simulink model "Final_Reciprocating_Simscape_Impedance_Hybrid_01_09_24_1_Pos"  (R2023b)
settings: Solver=VariableStepAuto  StartTime=0.0  StopTime=0.5  RelTol=1e-3
values from neighbouring files (symbols this model uses):
  d1 = 0    [FFFB_PosForce_ME1.m]    (also in FFFB_PosForce_ME2.m; FFFB_Posarbitary_actual_Mass.m; FFFB_arbitary_actual_Mass.m; Kin_sol_Pos2.m)
  d2 = 0    [FFFB_PosForce_ME1.m]    (also in FFFB_PosForce_ME2.m; FFFB_Posarbitary_actual_Mass.m; FFFB_arbitary_actual_Mass.m; Kin_sol_Pos2.m)
  k1 = 20    [FFFB_PosForce_ME1.m]    (also in FFFB_PosForce_ME2.m; FFFB_Posarbitary_actual_Mass.m; FFFB_arbitary_actual_Mass.m; KinAnimation_plot.m = double(a11*cos(f)*cos(t1+t2)-b11*sin(f)*sin(t1+t2)+P31(1)))
  k2 = 4    [FFFB_PosForce_ME1.m]    (also in FFFB_PosForce_ME2.m; FFFB_Posarbitary_actual_Mass.m; FFFB_arbitary_actual_Mass.m; KinAnimation_plot.m = double(a11*cos(f)*sin(t1+t2)+b11*sin(f)*cos(t1+t2)+P31(2)))
  Kd = 0.5    [FFFB_PosForce_ME.m]    (also in FFFB_PosForce_ME1.m = 2.8284; FFFB_PosForce_ME2.m = 2.8284; FFFB_Posarbitary_actual_Mass.m = 2.8284; FFFB_arbitary_actual_Mass.m = 2.8284)
  Kd1 = 1    [FFFB_PosForce_ME.m]    (also in FFFB_PosForce_ME1.m = 141.42; FFFB_PosForce_ME2.m = 141.42; FFFB_Posarbitary_actual_Mass.m = 141.42; FFFB_arbitary_actual_Mass.m = 141.42)
  Kd2 = 110    [FFFB_PosForce_ME1.m]    (also in FFFB_PosForce_ME2.m; FFFB_Posarbitary_actual_Mass.m; FFFB_arbitary_actual_Mass.m; Kin_sol_Pos2.m)
  Kp = 16    [FFFB_PosForce_ME.m]    (also in FFFB_PosForce_ME1.m = 2; FFFB_PosForce_ME2.m = 2; FFFB_Posarbitary_actual_Mass.m = 2; FFFB_arbitary_actual_Mass.m = 2)
  Kp1 = 10    [FFFB_PosForce_ME.m]    (also in FFFB_PosForce_ME1.m = 5000; FFFB_PosForce_ME2.m = 5000; FFFB_Posarbitary_actual_Mass.m = 5000; FFFB_arbitary_actual_Mass.m = 5000)
  Kp2 = 10000    [FFFB_PosForce_ME1.m]    (also in FFFB_PosForce_ME2.m; FFFB_Posarbitary_actual_Mass.m; FFFB_arbitary_actual_Mass.m; Kin_Trajectory_23_09_24.m)
  m1 = 0.6562    [FFFB_PosForce_ME1.m]    (also in FFFB_PosForce_ME2.m; FFFB_Posarbitary_actual_Mass.m; FFFB_arbitary_actual_Mass.m; Kin_sol_Pos2.m)
  m2 = 0.1355    [FFFB_PosForce_ME1.m]    (also in FFFB_PosForce_ME2.m; FFFB_Posarbitary_actual_Mass.m; FFFB_arbitary_actual_Mass.m; Kin_sol_Pos2.m)
  m3 = 0.1336    [FFFB_PosForce_ME1.m]    (also in FFFB_PosForce_ME2.m; FFFB_Posarbitary_actual_Mass.m; FFFB_arbitary_actual_Mass.m; Kin_sol_Pos2.m)
  N = [-y1+y3;-x3+x1]    [Contact.m]
  P = [X2';Y2';F2']    [FFFB_PosForce_ME.m]    (also in FFFB_PosForce_ME1.m = [X;Y;F_]; FFFB_PosForce_ME2.m = [X;Y;F_]; FFFB_Posarbitary_actual_Mass.m = [X;Y;F_]; FFFB_arbitary_actual_Mass.m = [X;Y;F_])
  Pd = [Xd2';Yd2';Fd2']    [FFFB_PosForce_ME.m]    (also in FFFB_PosForce_ME1.m = [Xd;Yd;Fd_]; FFFB_PosForce_ME2.m = [Xd;Yd;Fd_]; FFFB_Posarbitary_actual_Mass.m = [Xd;Yd;Fd_]; FFFB_arbitary_actual_Mass.m = [Xd;Yd;Fd_])
  Pdd = [Xdd2';Ydd2';Fdd2']    [FFFB_PosForce_ME.m]    (also in FFFB_PosForce_ME1.m = [Xdd;Ydd;Fdd_]; FFFB_PosForce_ME2.m = [Xdd;Ydd;Fdd_]; FFFB_Posarbitary_actual_Mass.m = [Xdd;Ydd;Fdd_]; FFFB_arbitary_actual_Mass.m = [Xdd;Ydd;Fdd_])
  X = 0.65    [Contact.m]    (also in FFFB_PosForce_ME.m = [X0',X1',X2']; FFFB_PosForce_ME1.m = [X2']; FFFB_PosForce_ME2.m = [X110,X2']; FFFB_Posarbitary_actual_Mass.m = [X110])
  Y = [Y0',Y1',Y2']    [FFFB_PosForce_ME.m]    (also in FFFB_PosForce_ME1.m = [Y2']; FFFB_PosForce_ME2.m = [Y110,Y2']; FFFB_Posarbitary_actual_Mass.m = [Y110]; FFFB_arbitary_actual_Mass.m = [Y2'])
undefined symbols (not defined in the file or in its folder): Ang, Z
libraries: sm_lib x24, nesl_utility x8, robotcorelib x1
settings Model: Creator=Dell  LastModifiedBy=91996

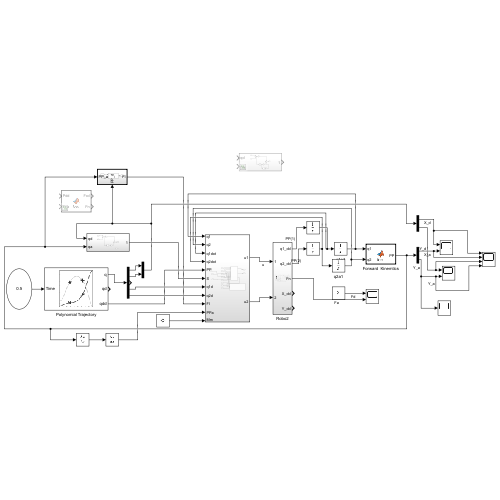
[thumbnail: Simulink's stored preview of the top-level diagram]
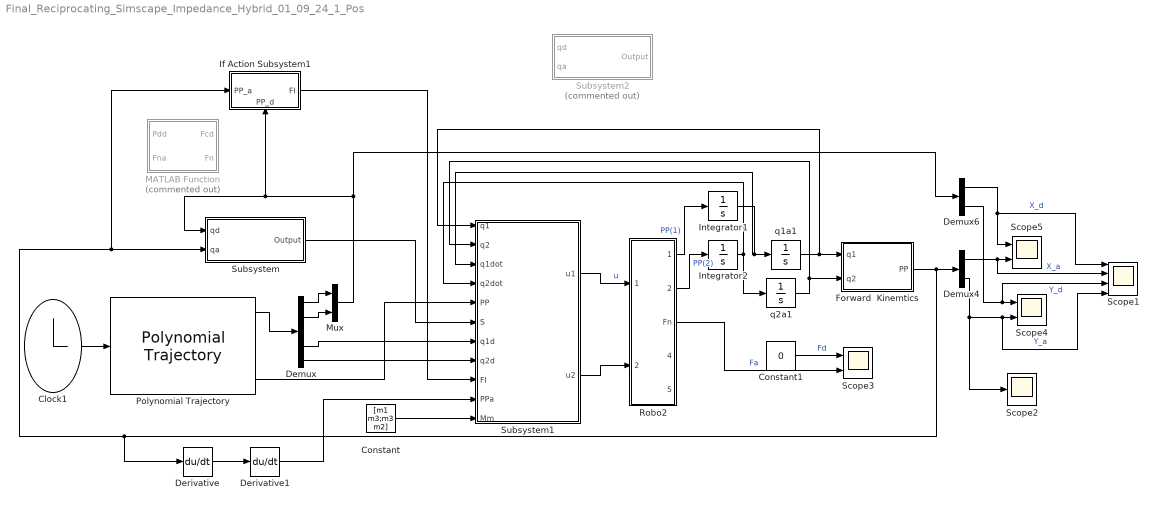
== system Final_Reciprocating_Simscape_Impedance_Hybrid_01_09_24_1_Pos ==
  Clock1 : Clock
  Constant : Constant  Value=[m1 m3;m3 m2]
  Constant1 : Constant  Value=0
  Demux : Demux  Outputs=5
  Demux4 : Demux  Outputs=2
  Demux6 : Demux  Outputs=2
  Derivative : Derivative
  Derivative1 : Derivative
  Forward  Kinemtics : MATLAB Function  TreatAsAtomicUnit=on
  If Action Subsystem1 : Subsystem  TreatAsAtomicUnit=on
      settings: PortSchema="{\"entries\":[{\"content\":{\"sides\":[{\"content\":{\"connectorIds\":[\"In1\"]},\"type\":\"ConnectorPlacement.EquallySpacedRectSide\",\"uuid\":\"1e1d39c2-5702-473c-8ff2-00e3ecdbae4f\"},{\"content\":{\"connectorIds\":[\"Out1\"],\"side\":\"RIGHT\"},\"type\":\"ConnectorPlacement.EquallySpacedRectSide\",\"uuid\":\"10dad59f-0c61-4f22-9a2f-e457bf203a4d\"},{\"content\":{\"side\":\"TOP\"},\"type\":\"ConnectorPlacement.EquallySpacedRectSide\",\"uuid\":\"73681e73-202a-4d7d-b740-7ea843c38ff3\"},{\"content\":{\"connectorIds\":[\"In2\"],\"side\":\"BOTTOM\"},\"type\":\"ConnectorPlacement.EquallySpacedRectSide\",\"uuid\":\"79dff506-e525-4b5b-bab4-76a6fcb6b4b4\"}]},\"type\":\"ConnectorPlacement.EquallySpacedConnector\",\"uuid\":\"cf80a0f8-aca3-4fef-8b76-fcb484b4ac5f\"}],\"packageUris\":[\"http://schema.mathworks.com/mf0/Connector/R2020b\"],\"version\":\"1.0\"}"
  Integrator1 : Integrator
  Integrator2 : Integrator
  MATLAB Function : MATLAB Function  Commented=on  TreatAsAtomicUnit=on
  Mux : Mux  Inputs=2
  Polynomial Trajectory : robotcorelib/Polynomial Trajectory  WaypointSource=Internal  Waypoints=[P;Ang]  TimePoints=T  TimeInterval=[ 1, 4 ]  Method=Quintic Polynomial  ParameterSource=Internal  VelocityBoundaryCondition=[Pd;Ang]  AccelerationBoundaryCondition=[Pdd;Ang]  SimulateUsing=Interpreted execution
  Robo2 : Subsystem
  Scope1 : Scope  NumInputPorts=4
  Scope2 : Scope
  Scope3 : Scope  NumInputPorts=2
  Scope4 : Scope  NumInputPorts=2
  Scope5 : Scope  NumInputPorts=2
  Subsystem : Subsystem
  Subsystem1 : Subsystem
  Subsystem2 : Subsystem  Commented=on
  q1a1 : Integrator  InitialCondition=0.3963
  q2a1 : Integrator  InitialCondition=-1.5800
  wires:
  Robo2/1(q1_dd) -> Integrator1/1  "PP(1)"
  Demux/5 -> Subsystem1/8(q2d)
  Integrator1/1 -> Subsystem1/3(q1dot), q1a1/1
  Demux/4 -> Subsystem1/7(q1d)
  Robo2/3(Fn) -> Scope3/2  "Fa"
  Polynomial Trajectory/1 -> Demux/1
  Demux/2 -> Mux/2
  Demux/1 -> Mux/1
  Polynomial Trajectory/3 -> Subsystem1/5(PP)
  Subsystem/1(Output) -> Subsystem1/6(S)
  Subsystem1/1(u1) -> Robo2/1(Input)  "u"
  Demux4/2 -> Scope2/1, Scope1/4, Scope4/2  "Y_a"
  Constant1/1 -> Scope3/1  "Fd"
  Subsystem1/2(u2) -> Robo2/2(Input1)
  Demux6/1 -> Scope5/1, Scope1/1  "X_d"
  Robo2/2(q2_dd) -> Integrator2/1  "PP(2)"
  Clock1/1 -> Polynomial Trajectory/1
  Mux/1 -> Demux6/1, Subsystem/1(qd), If Action Subsystem1/2(PP_d)
  Demux6/2 -> Scope1/3, Scope4/1  "Y_d"
  Integrator2/1 -> q2a1/1, Subsystem1/4(q2dot)
  q1a1/1 -> Forward  Kinemtics/1(q1), Subsystem1/1(q1)
  Forward  Kinemtics/1(PP) -> Derivative/1, If Action Subsystem1/1(PP_a), Subsystem/2(qa), Demux4/1
  Demux4/1 -> Scope1/2, Scope5/2  "X_a"
  q2a1/1 -> Forward  Kinemtics/2(q2), Subsystem1/2(q2)
  If Action Subsystem1/1(FI) -> Subsystem1/9(FI)
  Constant/1 -> Subsystem1/11(Mm)
  Derivative/1 -> Derivative1/1
  Derivative1/1 -> Subsystem1/10(PPa)

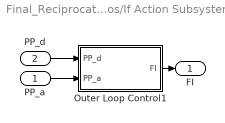
== system Final_Reciprocating_Simscape_Impedance_Hybrid_01_09_24_1_Pos/If Action Subsystem1 ==
  PP_a : Inport
  PP_d : Inport  Port=2
  Outer Loop Control1 : Subsystem
  FI : Outport
  wires:
  PP_d/1 -> Outer Loop Control1/1(PP_d)
  Outer Loop Control1/1(FI) -> FI/1
  PP_a/1 -> Outer Loop Control1/2(PP_a)

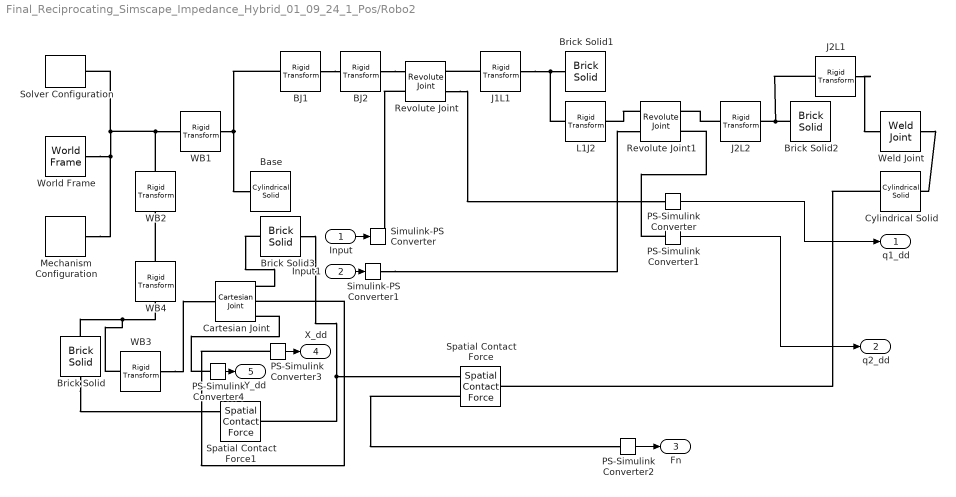
== system Final_Reciprocating_Simscape_Impedance_Hybrid_01_09_24_1_Pos/Robo2 ==
  Input : Inport
  Input1 : Inport  Port=2
  BJ1 : sm_lib/Frames and Transforms/Rigid Transform  TranslationMethod=StandardAxis  TranslationStandardOffset=0.25  TranslationStandardOffsetUnits=m  TranslationStandardAxis=+Z  TranslationCartesianOffset=[0 0 0]  TranslationCartesianOffsetUnits=m  TranslationROffset=0  TranslationROffsetUnits=m  TranslationZOffset=0  TranslationZOffsetUnits=m  TranslationThetaOffset=0  TranslationThetaOffsetUnits=deg  RotationMethod=StandardAxis  RotationAngleUnits=deg  RotationStandardAxis=+X  RotationAngle=90  RotationArbitraryAxis=[0 0 1]  FollAlignAxisA=+X  BaseAlignAxisA=+Y  FollAlignAxisB=+Y  BaseAlignAxisB=+Z  RotationSequenceAxes=FollowerAxes  RotationSequence=XYX  RotationSequenceAngles=[0 0 0]  RotationSequenceAnglesUnits=deg  RotationMatrix=[1 0 0; 0 1 0; 0 0 1]  Quaternion=[1 0 0 0]
  BJ2 : sm_lib/Frames and Transforms/Rigid Transform  TranslationMethod=None  TranslationStandardOffset=0  TranslationStandardOffsetUnits=m  TranslationStandardAxis=+Z  TranslationCartesianOffset=[0 0 0]  TranslationCartesianOffsetUnits=m  TranslationROffset=0  TranslationROffsetUnits=m  TranslationZOffset=0  TranslationZOffsetUnits=m  TranslationThetaOffset=0  TranslationThetaOffsetUnits=deg  RotationMethod=StandardAxis  RotationAngleUnits=rad  RotationStandardAxis=+Z  RotationAngle=0.3963  RotationArbitraryAxis=[0 0 1]  FollAlignAxisA=+X  BaseAlignAxisA=+Y  FollAlignAxisB=+Y  BaseAlignAxisB=+Z  RotationSequenceAxes=FollowerAxes  RotationSequence=XYX  RotationSequenceAngles=[0 0 0]  RotationSequenceAnglesUnits=deg  RotationMatrix=[1 0 0; 0 1 0; 0 0 1]  Quaternion=[1 0 0 0]
  Base : sm_lib/Body Elements/Cylindrical Solid  GraphicAmbientColor=[0.15 0.15 0.15 1.0]  BasedOnType=Density  CenterOfMass=[0 0 0]  CenterOfMassUnits=m  GraphicDiffuseColor=[0.5 0.5 0.5]  CylinderLength=0.5  CylinderLengthUnits=m  CylinderRadius=0.02  CylinderRadiusUnits=m  Density=10000  DensityUnits=kg/m^3  DoExposeReferenceFrame=on  GraphicEmissiveColor=[0.0 0.0 0.0 1.0]  ExportEntireGeometry=off  SerializedFrames=<Frames/>  MarkerShape=Sphere  MarkerSize=10  GraphicType=FromGeometry  InertiaType=CalculateFromGeometry  Mass=1  MassUnits=kg  MomentsOfInertia=[1 1 1]  MomentsOfInertiaUnits=kg*m^2  GraphicOpacity=1.0  ProductsOfInertia=[0 0 0]  ProductsOfInertiaUnits=kg*m^2  GraphicShininess=75  GraphicSpecularColor=[0.5 0.5 0.5 1.0]  GraphicVisPropType=SimpleVisualProperties
  Brick Solid : sm_lib/Body Elements/Brick Solid  GraphicAmbientColor=[0.15 0.15 0.15 1.0]  BasedOnType=Density  BrickDimensions=[1 0.02 0.02]  BrickDimensionsUnits=m  CenterOfMass=[0 0 0]  CenterOfMassUnits=m  GraphicDiffuseColor=[0.5 0.5 0.5]  Density=10000  DensityUnits=kg/m^3  DoExposeReferenceFrame=on  GraphicEmissiveColor=[0.0 0.0 0.0 1.0]  ExportEntireGeometry=on  SerializedFrames=<Frames/>  MarkerShape=Sphere  MarkerSize=10  GraphicType=FromGeometry  InertiaType=CalculateFromGeometry  Mass=1  MassUnits=kg  MomentsOfInertia=[1 1 1]  MomentsOfInertiaUnits=kg*m^2  GraphicOpacity=1.0  ProductsOfInertia=[0 0 0]  ProductsOfInertiaUnits=kg*m^2  GraphicShininess=75  GraphicSpecularColor=[0.5 0.5 0.5 1.0]  GraphicVisPropType=SimpleVisualProperties
  Brick Solid1 : sm_lib/Body Elements/Brick Solid  GraphicAmbientColor=[0.15 0.15 0.15 1.0]  BasedOnType=Density  BrickDimensions=[0.5 0.02 0.02]  BrickDimensionsUnits=m  CenterOfMass=[0 0 0]  CenterOfMassUnits=m  GraphicDiffuseColor=[0.2 0.2 1.0]  Density=7800  DensityUnits=kg/m^3  DoExposeReferenceFrame=on  GraphicEmissiveColor=[0.0 0.0 0.0 1.0]  ExportEntireGeometry=off  SerializedFrames=<Frames/>  MarkerShape=Sphere  MarkerSize=10  GraphicType=FromGeometry  InertiaType=CalculateFromGeometry  Mass=1  MassUnits=kg  MomentsOfInertia=[1 1 1]  MomentsOfInertiaUnits=kg*m^2  GraphicOpacity=1.0  ProductsOfInertia=[0 0 0]  ProductsOfInertiaUnits=kg*m^2  GraphicShininess=75  GraphicSpecularColor=[0.5 0.5 0.5 1.0]  GraphicVisPropType=SimpleVisualProperties
  Brick Solid2 : sm_lib/Body Elements/Brick Solid  GraphicAmbientColor=[0.15 0.15 0.15 1.0]  BasedOnType=Density  BrickDimensions=[0.5 0.02 0.02]  BrickDimensionsUnits=m  CenterOfMass=[0 0 0]  CenterOfMassUnits=m  GraphicDiffuseColor=[0.0 0.8 0.2]  Density=7800  DensityUnits=kg/m^3  DoExposeReferenceFrame=on  GraphicEmissiveColor=[0.0 0.0 0.0 1.0]  ExportEntireGeometry=off  SerializedFrames=<Frames/>  MarkerShape=Sphere  MarkerSize=10  GraphicType=FromGeometry  InertiaType=CalculateFromGeometry  Mass=1  MassUnits=kg  MomentsOfInertia=[1 1 1]  MomentsOfInertiaUnits=kg*m^2  GraphicOpacity=1.0  ProductsOfInertia=[0 0 0]  ProductsOfInertiaUnits=kg*m^2  GraphicShininess=75  GraphicSpecularColor=[0.5 0.5 0.5 1.0]  GraphicVisPropType=SimpleVisualProperties
  Brick Solid3 : sm_lib/Body Elements/Brick Solid  GraphicAmbientColor=[0.15 0.15 0.15 1.0]  BasedOnType=Density  BrickDimensions=[0.2 0.02 0.2]  BrickDimensionsUnits=m  CenterOfMass=[0 0 0]  CenterOfMassUnits=m  GraphicDiffuseColor=[1.0 0.2 0.2]  Density=2000  DensityUnits=kg/m^3  DoExposeReferenceFrame=on  GraphicEmissiveColor=[0.0 0.0 0.0 1.0]  ExportEntireGeometry=on  SerializedFrames=<Frames/>  MarkerShape=Sphere  MarkerSize=10  GraphicType=FromGeometry  InertiaType=CalculateFromGeometry  Mass=1  MassUnits=kg  MomentsOfInertia=[1 1 1]  MomentsOfInertiaUnits=kg*m^2  GraphicOpacity=1.0  ProductsOfInertia=[0 0 0]  ProductsOfInertiaUnits=kg*m^2  GraphicShininess=75  GraphicSpecularColor=[0.5 0.5 0.5 1.0]  GraphicVisPropType=SimpleVisualProperties
  Cartesian Joint : sm_lib/Joints/Cartesian Joint  JointMode=Normal  SenseConstraintForce=off  SenseConstraintForceX=off  SenseConstraintForceY=off  SenseConstraintForceZ=off  SenseConstraintTorque=off  SenseConstraintTorqueX=off  SenseConstraintTorqueY=off  SenseConstraintTorqueZ=off  SenseTotalForce=off  SenseTotalForceX=off  SenseTotalForceY=off  SenseTotalForceZ=off  SenseTotalTorque=off  SenseTotalTorqueX=off  SenseTotalTorqueY=off  SenseTotalTorqueZ=off  CompositeWrenchDir=FollowerOnBase  CompositeWrenchFrame=BaseFrame  PxEquilibriumPosition=0  PxEquilibriumPositionUnits=m  PxSpringStiffness=0  PxSpringStiffnessUnits=N/m  PxDampingCoefficient=0  PxDampingCoefficientUnits=N/(m/s)  PxTorqueActuationMode=NoTorque  PxMotionActuationMode=ComputedMotion  PxSensePosition=off  PxSenseVelocity=off  PxSenseAcceleration=on  PxSenseTorqueForce=off  PxSenseLowerLimitTorqueForce=off  PxSenseUpperLimitTorqueForce=off  PxLowerLimitSpecify=off  PxLowerLimitBound=-1  PxLowerLimitBoundUnits=m  PxLowerLimitStiffness=1e6  PxLowerLimitStiffnessUnits=N/m  PxLowerLimitDamping=1e3  PxLowerLimitDampingUnits=N/(m/s)  PxLowerLimitTransitionRegionWidth=1e-4  PxLowerLimitTransitionRegionWidthUnits=m  PxUpperLimitSpecify=off  PxUpperLimitBound=1  PxUpperLimitBoundUnits=m  PxUpperLimitStiffness=1e6  PxUpperLimitStiffnessUnits=N/m  PxUpperLimitDamping=1e3  PxUpperLimitDampingUnits=N/(m/s)  PxUpperLimitTransitionRegionWidth=1e-4  PxUpperLimitTransitionRegionWidthUnits=m  PxPositionTargetSpecify=off  PxPositionTargetPriority=High  PxPositionTargetValue=0  PxPositionTargetValueUnits=m  PxVelocityTargetSpecify=off  PxVelocityTargetPriority=High  PxVelocityTargetValue=0  PxVelocityTargetValueUnits=m/s  PyEquilibriumPosition=0  PyEquilibriumPositionUnits=m  PySpringStiffness=0  PySpringStiffnessUnits=N/m  PyDampingCoefficient=0  PyDampingCoefficientUnits=N/(m/s)  PyTorqueActuationMode=NoTorque  PyMotionActuationMode=ComputedMotion  PySensePosition=off  PySenseVelocity=off  PySenseAcceleration=off  PySenseTorqueForce=off  PySenseLowerLimitTorqueForce=off  PySenseUpperLimitTorqueForce=off  PyLowerLimitSpecify=off  PyLowerLimitBound=-1  PyLowerLimitBoundUnits=m  PyLowerLimitStiffness=1e6  PyLowerLimitStiffnessUnits=N/m  PyLowerLimitDamping=1e3  PyLowerLimitDampingUnits=N/(m/s)  PyLowerLimitTransitionRegionWidth=1e-4  PyLowerLimitTransitionRegionWidthUnits=m  PyUpperLimitSpecify=off  PyUpperLimitBound=1  PyUpperLimitBoundUnits=m  PyUpperLimitStiffness=1e6  PyUpperLimitStiffnessUnits=N/m  PyUpperLimitDamping=1e3  PyUpperLimitDampingUnits=N/(m/s)  PyUpperLimitTransitionRegionWidth=1e-4  PyUpperLimitTransitionRegionWidthUnits=m  PyPositionTargetSpecify=off  PyPositionTargetPriority=High  PyPositionTargetValue=0  PyPositionTargetValueUnits=m  PyVelocityTargetSpecify=off  PyVelocityTargetPriority=High  PyVelocityTargetValue=0  PyVelocityTargetValueUnits=m/s  PzEquilibriumPosition=0  PzEquilibriumPositionUnits=m  PzSpringStiffness=0  PzSpringStiffnessUnits=N/m  PzDampingCoefficient=0  PzDampingCoefficientUnits=N/(m/s)  PzTorqueActuationMode=NoTorque  PzMotionActuationMode=ComputedMotion  PzSensePosition=off  PzSenseVelocity=off  PzSenseAcceleration=on  PzSenseTorqueForce=off  PzSenseLowerLimitTorqueForce=off  PzSenseUpperLimitTorqueForce=off  PzLowerLimitSpecify=off  PzLowerLimitBound=-1  PzLowerLimitBoundUnits=m  PzLowerLimitStiffness=1e6  PzLowerLimitStiffnessUnits=N/m  PzLowerLimitDamping=1e3  PzLowerLimitDampingUnits=N/(m/s)  PzLowerLimitTransitionRegionWidth=1e-4  PzLowerLimitTransitionRegionWidthUnits=m  PzUpperLimitSpecify=off  PzUpperLimitBound=1  PzUpperLimitBoundUnits=m  PzUpperLimitStiffness=1e6  PzUpperLimitStiffnessUnits=N/m  PzUpperLimitDamping=1e3  PzUpperLimitDampingUnits=N/(m/s)  PzUpperLimitTransitionRegionWidth=1e-4  PzUpperLimitTransitionRegionWidthUnits=m  PzPositionTargetSpecify=off  PzPositionTargetPriority=High  PzPositionTargetValue=0  PzPositionTargetValueUnits=m  PzVelocityTargetSpecify=off  PzVelocityTargetPriority=High  PzVelocityTargetValue=0  PzVelocityTargetValueUnits=m/s
  Cylindrical Solid : sm_lib/Body Elements/Cylindrical Solid  GraphicAmbientColor=[0.15 0.15 0.15 1.0]  BasedOnType=Density  CenterOfMass=[0 0 0]  CenterOfMassUnits=m  GraphicDiffuseColor=[0.5 0.5 0.5]  CylinderLength=0.02  CylinderLengthUnits=m  CylinderRadius=0.01  CylinderRadiusUnits=m  Density=7800  DensityUnits=kg/m^3  DoExposeReferenceFrame=on  GraphicEmissiveColor=[0.0 0.0 0.0 1.0]  ExportEntireGeometry=on  SerializedFrames=<Frames/>  MarkerShape=Sphere  MarkerSize=10  GraphicType=FromGeometry  InertiaType=CalculateFromGeometry  Mass=1  MassUnits=kg  MomentsOfInertia=[1 1 1]  MomentsOfInertiaUnits=kg*m^2  GraphicOpacity=1.0  ProductsOfInertia=[0 0 0]  ProductsOfInertiaUnits=kg*m^2  GraphicShininess=75  GraphicSpecularColor=[0.5 0.5 0.5 1.0]  GraphicVisPropType=SimpleVisualProperties
  J1L1 : sm_lib/Frames and Transforms/Rigid Transform  TranslationMethod=StandardAxis  TranslationStandardOffset=0.25  TranslationStandardOffsetUnits=m  TranslationStandardAxis=+X  TranslationCartesianOffset=[0 0 0]  TranslationCartesianOffsetUnits=m  TranslationROffset=0  TranslationROffsetUnits=m  TranslationZOffset=0  TranslationZOffsetUnits=m  TranslationThetaOffset=0  TranslationThetaOffsetUnits=deg  RotationMethod=None  RotationAngleUnits=deg  RotationStandardAxis=+Z  RotationAngle=0.0  RotationArbitraryAxis=[0 0 1]  FollAlignAxisA=+X  BaseAlignAxisA=+Y  FollAlignAxisB=+Y  BaseAlignAxisB=+Z  RotationSequenceAxes=FollowerAxes  RotationSequence=XYX  RotationSequenceAngles=[0 0 0]  RotationSequenceAnglesUnits=deg  RotationMatrix=[1 0 0; 0 1 0; 0 0 1]  Quaternion=[1 0 0 0]
  J2L1 : sm_lib/Frames and Transforms/Rigid Transform  TranslationMethod=StandardAxis  TranslationStandardOffset=(0.5)/2  TranslationStandardOffsetUnits=m  TranslationStandardAxis=+X  TranslationCartesianOffset=[0 0 0]  TranslationCartesianOffsetUnits=m  TranslationROffset=0  TranslationROffsetUnits=m  TranslationZOffset=0  TranslationZOffsetUnits=m  TranslationThetaOffset=0  TranslationThetaOffsetUnits=deg  RotationMethod=None  RotationAngleUnits=deg  RotationStandardAxis=+Z  RotationAngle=0.0  RotationArbitraryAxis=[0 0 1]  FollAlignAxisA=+X  BaseAlignAxisA=+Y  FollAlignAxisB=+Y  BaseAlignAxisB=+Z  RotationSequenceAxes=FollowerAxes  RotationSequence=XYX  RotationSequenceAngles=[0 0 0]  RotationSequenceAnglesUnits=deg  RotationMatrix=[1 0 0; 0 1 0; 0 0 1]  Quaternion=[1 0 0 0]
  J2L2 : sm_lib/Frames and Transforms/Rigid Transform  TranslationMethod=StandardAxis  TranslationStandardOffset=(0.5)/2  TranslationStandardOffsetUnits=m  TranslationStandardAxis=+X  TranslationCartesianOffset=[0 0 0]  TranslationCartesianOffsetUnits=m  TranslationROffset=0  TranslationROffsetUnits=m  TranslationZOffset=0  TranslationZOffsetUnits=m  TranslationThetaOffset=0  TranslationThetaOffsetUnits=deg  RotationMethod=None  RotationAngleUnits=deg  RotationStandardAxis=+Z  RotationAngle=0.0  RotationArbitraryAxis=[0 0 1]  FollAlignAxisA=+X  BaseAlignAxisA=+Y  FollAlignAxisB=+Y  BaseAlignAxisB=+Z  RotationSequenceAxes=FollowerAxes  RotationSequence=XYX  RotationSequenceAngles=[0 0 0]  RotationSequenceAnglesUnits=deg  RotationMatrix=[1 0 0; 0 1 0; 0 0 1]  Quaternion=[1 0 0 0]
  L1J2 : sm_lib/Frames and Transforms/Rigid Transform  TranslationMethod=StandardAxis  TranslationStandardOffset=0.25  TranslationStandardOffsetUnits=m  TranslationStandardAxis=+X  TranslationCartesianOffset=[0 0 0]  TranslationCartesianOffsetUnits=m  TranslationROffset=0  TranslationROffsetUnits=m  TranslationZOffset=0  TranslationZOffsetUnits=m  TranslationThetaOffset=0  TranslationThetaOffsetUnits=deg  RotationMethod=StandardAxis  RotationAngleUnits=rad  RotationStandardAxis=+Z  RotationAngle=-1.5800  RotationArbitraryAxis=[0 0 1]  FollAlignAxisA=+X  BaseAlignAxisA=+Y  FollAlignAxisB=+Y  BaseAlignAxisB=+Z  RotationSequenceAxes=FollowerAxes  RotationSequence=XYX  RotationSequenceAngles=[0 0 0]  RotationSequenceAnglesUnits=deg  RotationMatrix=[1 0 0; 0 1 0; 0 0 1]  Quaternion=[1 0 0 0]
  Mechanism Configuration : sm_lib/Utilities/Mechanism Configuration  UniformGravity=Constant  GravityVector=[0 0 -9.80665]  GravityVectorUnits=m/s^2  LinearizationDelta=0.001  JointModeTransitionNonlinearIterations=2
  PS-Simulink Converter{,1..4} (5 alike) : nesl_utility/PS-Simulink Converter  PhysicalDomain=network_engine_domain  SubClassName=ps_output  LeftPortType=input  RightPortType=output  PseudoPeriodic=off  Frequencies=[]  VectorFormat=inherit  Unit=inherit  AffineConversion=off
  Revolute Joint : sm_lib/Joints/Revolute Joint  JointMode=Normal  SenseConstraintForce=off  SenseConstraintForceX=off  SenseConstraintForceY=off  SenseConstraintForceZ=off  SenseConstraintTorque=off  SenseConstraintTorqueX=off  SenseConstraintTorqueY=off  SenseConstraintTorqueZ=off  SenseTotalForce=off  SenseTotalForceX=off  SenseTotalForceY=off  SenseTotalForceZ=off  SenseTotalTorque=off  SenseTotalTorqueX=off  SenseTotalTorqueY=off  SenseTotalTorqueZ=off  CompositeWrenchDir=FollowerOnBase  CompositeWrenchFrame=BaseFrame  EquilibriumPosition=0  EquilibriumPositionUnits=deg  SpringStiffness=0  SpringStiffnessUnits=N*m/deg  DampingCoefficient=0  DampingCoefficientUnits=N*m/(deg/s)  TorqueActuationMode=InputTorque  MotionActuationMode=ComputedMotion  SensePosition=off  SenseVelocity=off  SenseAcceleration=on  SenseTorqueForce=off  SenseLowerLimitTorqueForce=off  SenseUpperLimitTorqueForce=off  LowerLimitSpecify=off  LowerLimitBound=-90  LowerLimitBoundUnits=deg  LowerLimitStiffness=1e4  LowerLimitStiffnessUnits=N*m/deg  LowerLimitDamping=10  LowerLimitDampingUnits=N*m/(deg/s)  LowerLimitTransitionRegionWidth=0.1  LowerLimitTransitionRegionWidthUnits=deg  UpperLimitSpecify=off  UpperLimitBound=90  UpperLimitBoundUnits=deg  UpperLimitStiffness=1e4  UpperLimitStiffnessUnits=N*m/deg  UpperLimitDamping=10  UpperLimitDampingUnits=N*m/(deg/s)  UpperLimitTransitionRegionWidth=0.1  UpperLimitTransitionRegionWidthUnits=deg  PositionTargetSpecify=off  PositionTargetPriority=High  PositionTargetValue=0  PositionTargetValueUnits=deg  VelocityTargetSpecify=off  VelocityTargetPriority=High  VelocityTargetValue=0  VelocityTargetValueUnits=deg/s
  Revolute Joint1 : sm_lib/Joints/Revolute Joint  JointMode=Normal  SenseConstraintForce=off  SenseConstraintForceX=off  SenseConstraintForceY=off  SenseConstraintForceZ=off  SenseConstraintTorque=off  SenseConstraintTorqueX=off  SenseConstraintTorqueY=off  SenseConstraintTorqueZ=off  SenseTotalForce=off  SenseTotalForceX=off  SenseTotalForceY=off  SenseTotalForceZ=off  SenseTotalTorque=off  SenseTotalTorqueX=off  SenseTotalTorqueY=off  SenseTotalTorqueZ=off  CompositeWrenchDir=FollowerOnBase  CompositeWrenchFrame=BaseFrame  EquilibriumPosition=0  EquilibriumPositionUnits=deg  SpringStiffness=0  SpringStiffnessUnits=N*m/deg  DampingCoefficient=0  DampingCoefficientUnits=N*m/(deg/s)  TorqueActuationMode=InputTorque  MotionActuationMode=ComputedMotion  SensePosition=off  SenseVelocity=off  SenseAcceleration=on  SenseTorqueForce=off  SenseLowerLimitTorqueForce=off  SenseUpperLimitTorqueForce=off  LowerLimitSpecify=off  LowerLimitBound=-90  LowerLimitBoundUnits=deg  LowerLimitStiffness=1e4  LowerLimitStiffnessUnits=N*m/deg  LowerLimitDamping=10  LowerLimitDampingUnits=N*m/(deg/s)  LowerLimitTransitionRegionWidth=0.1  LowerLimitTransitionRegionWidthUnits=deg  UpperLimitSpecify=off  UpperLimitBound=90  UpperLimitBoundUnits=deg  UpperLimitStiffness=1e4  UpperLimitStiffnessUnits=N*m/deg  UpperLimitDamping=10  UpperLimitDampingUnits=N*m/(deg/s)  UpperLimitTransitionRegionWidth=0.1  UpperLimitTransitionRegionWidthUnits=deg  PositionTargetSpecify=off  PositionTargetPriority=High  PositionTargetValue=0  PositionTargetValueUnits=deg  VelocityTargetSpecify=off  VelocityTargetPriority=High  VelocityTargetValue=0  VelocityTargetValueUnits=deg/s
  Simulink-PS Converter : nesl_utility/Simulink-PS Converter  PhysicalDomain=network_engine_domain  SubClassName=ps_input  LeftPortType=input  RightPortType=output  PseudoPeriodic=off  Frequencies=[]  NoiseDistribution=none  NoiseParameters=[]  Unit=N*m  AffineConversion=off  FilteringAndDerivatives=provide  SimscapeFilterOrder=1  InputFilterTimeConstant=0.001  UdotUserProvided=0
  Simulink-PS Converter1 : nesl_utility/Simulink-PS Converter  PhysicalDomain=network_engine_domain  SubClassName=ps_input  LeftPortType=input  RightPortType=output  PseudoPeriodic=off  Frequencies=[]  NoiseDistribution=none  NoiseParameters=[]  Unit=N*m  AffineConversion=off  FilteringAndDerivatives=provide  SimscapeFilterOrder=1  InputFilterTimeConstant=0.001  UdotUserProvided=0
  Solver Configuration : nesl_utility/Solver Configuration  PhysicalDomain=network_engine_domain  SubClassName=solver  LeftPortType=input  RightPortType=generic  Tones=[]  Harmonics=[]  SimulateNoise=off  Profile=off  UseLocalSampling=off  EnableSwitchedLinearOptims=on  FrequencyDomain=off  UseCCode=off  RelTol=0.001  AbsTol=1e-06  MinStep=1e-09  ToWorkspace=off  RevertToSquareIcSolve=off  NumHomotopyIterations=100  PhasorMode=off  PhasorModeNumHarmonics=1  ConsistencySolver=NEWTON_XTOL_AFTER_FTOL  IndexReductionMethod=DerivativeReplacement  DoDC=off  ResidualTolerance=1e-09  ConsistencyTolSource=GLOBAL  ConsistencyAbsTol=0.001  ConsistencyRelTol=0.001  ConsistencyTolFactor=0.001  UseLocalSolver=off  LocalSolverChoice=NE_BACKWARD_EULER_ADVANCER  ResolveIndetEquations=on  FunctionEvalNumThread=1  LocalSolverSampleTime=0.001  DoFixedCost=off  MaxNonlinIter=3  MaxModeIter=2  ComputeImpulses=off  ImpulseIterations=2  LinearAlgebra=Sparse  LinearAlgebraNumThread=0  EquationFormulation=NE_TIME_EF  DelaysMemoryBudget=1024  AutomaticFiltering=on  FilteringTimeConstant=0.001  PartitionStorageMethod=AS_NEEDED  PartitionMemoryBudget=1024  PartitionMethod=FAST  MultibodyUseLocalSolver=off  MultibodyLocalSolverChoice=ODE1  MultibodyLocalSolverSampleTime=0.001
  Spatial Contact Force : sm_lib/Forces and Torques/Spatial Contact Force  SenseContactBaseRotation=off  SenseContactBaseTranslation=off  CoefficientOfDynamicFriction=0.3  CoefficientOfStaticFriction=0.5  NormalDamping=1e6  NormalDampingUnits=N/(m/s)  SenseContactSignal=off  NormalStiffness=1e6  NormalStiffnessUnits=N/m  FrictionalCriticalVelocity=1e-3  FrictionalCriticalVelocityUnits=m/s  ZeroCrossDetectContactStartAndEnd=off  SenseContactFollowerRotation=off  SenseContactFollowerTranslation=off  FrictionType=SmoothStickSlip  SenseFrictionalForceMagnitude=off  SenseNormalForceMagnitude=on  NormalForceType=SmoothSpringDamper  SenseNormalVelocity=off  SensePenetrationDepth=off  SenseSeparationDistance=off  SenseTangentialVelocity=off  NormalTransitionRegionWidth=1e-4  NormalTransitionRegionWidthUnits=m
  Spatial Contact Force1 : sm_lib/Forces and Torques/Spatial Contact Force  SenseContactBaseRotation=off  SenseContactBaseTranslation=off  CoefficientOfDynamicFriction=0.05  CoefficientOfStaticFriction=0.1  NormalDamping=1e6  NormalDampingUnits=N/(m/s)  SenseContactSignal=off  NormalStiffness=1e6  NormalStiffnessUnits=N/m  FrictionalCriticalVelocity=1e-3  FrictionalCriticalVelocityUnits=m/s  ZeroCrossDetectContactStartAndEnd=off  SenseContactFollowerRotation=off  SenseContactFollowerTranslation=off  FrictionType=SmoothStickSlip  SenseFrictionalForceMagnitude=off  SenseNormalForceMagnitude=on  NormalForceType=SmoothSpringDamper  SenseNormalVelocity=off  SensePenetrationDepth=off  SenseSeparationDistance=off  SenseTangentialVelocity=off  NormalTransitionRegionWidth=1e-4  NormalTransitionRegionWidthUnits=m
  WB1 : sm_lib/Frames and Transforms/Rigid Transform  TranslationMethod=Cartesian  TranslationStandardOffset=0  TranslationStandardOffsetUnits=m  TranslationStandardAxis=+Z  TranslationCartesianOffset=[0 0.25 0]  TranslationCartesianOffsetUnits=m  TranslationROffset=0  TranslationROffsetUnits=m  TranslationZOffset=0  TranslationZOffsetUnits=m  TranslationThetaOffset=0  TranslationThetaOffsetUnits=deg  RotationMethod=None  RotationAngleUnits=deg  RotationStandardAxis=+X  RotationAngle=90  RotationArbitraryAxis=[0 0 1]  FollAlignAxisA=+X  BaseAlignAxisA=+Y  FollAlignAxisB=+Y  BaseAlignAxisB=+Z  RotationSequenceAxes=FollowerAxes  RotationSequence=XYX  RotationSequenceAngles=[0 0 0]  RotationSequenceAnglesUnits=deg  RotationMatrix=[1 0 0; 0 1 0; 0 0 1]  Quaternion=[1 0 0 0]
  WB2 : sm_lib/Frames and Transforms/Rigid Transform  TranslationMethod=Cartesian  TranslationStandardOffset=0  TranslationStandardOffsetUnits=m  TranslationStandardAxis=+Z  TranslationCartesianOffset="[-0.5   -0.25  0.25 ]"  TranslationCartesianOffsetUnits=m  TranslationROffset=0  TranslationROffsetUnits=m  TranslationZOffset=0  TranslationZOffsetUnits=m  TranslationThetaOffset=0  TranslationThetaOffsetUnits=deg  RotationMethod=None  RotationAngleUnits=deg  RotationStandardAxis=+X  RotationAngle=90  RotationArbitraryAxis=[0 0 1]  FollAlignAxisA=+X  BaseAlignAxisA=+Y  FollAlignAxisB=+Y  BaseAlignAxisB=+Z  RotationSequenceAxes=FollowerAxes  RotationSequence=XYX  RotationSequenceAngles=[0 0 0]  RotationSequenceAnglesUnits=deg  RotationMatrix=[1 0 0; 0 1 0; 0 0 1]  Quaternion=[1 0 0 0]
  WB3 : sm_lib/Frames and Transforms/Rigid Transform  TranslationMethod=Cartesian  TranslationStandardOffset=0  TranslationStandardOffsetUnits=m  TranslationStandardAxis=+Z  TranslationCartesianOffset="[-0.24  0  -0.1-0.01 ]"  TranslationCartesianOffsetUnits=m  TranslationROffset=0  TranslationROffsetUnits=m  TranslationZOffset=0  TranslationZOffsetUnits=m  TranslationThetaOffset=0  TranslationThetaOffsetUnits=deg  RotationMethod=None  RotationAngleUnits=deg  RotationStandardAxis=+X  RotationAngle=90  RotationArbitraryAxis=[0 0 1]  FollAlignAxisA=+X  BaseAlignAxisA=+Y  FollAlignAxisB=+Y  BaseAlignAxisB=+Z  RotationSequenceAxes=FollowerAxes  RotationSequence=XYX  RotationSequenceAngles=[0 0 0]  RotationSequenceAnglesUnits=deg  RotationMatrix=[1 0 0; 0 1 0; 0 0 1]  Quaternion=[1 0 0 0]
  WB4 : sm_lib/Frames and Transforms/Rigid Transform  TranslationMethod=Cartesian  TranslationStandardOffset=0  TranslationStandardOffsetUnits=m  TranslationStandardAxis=+Z  TranslationCartesianOffset=[0,0,0.01 ]  TranslationCartesianOffsetUnits=m  TranslationROffset=0  TranslationROffsetUnits=m  TranslationZOffset=0  TranslationZOffsetUnits=m  TranslationThetaOffset=0  TranslationThetaOffsetUnits=deg  RotationMethod=None  RotationAngleUnits=deg  RotationStandardAxis=+X  RotationAngle=90  RotationArbitraryAxis=[0 0 1]  FollAlignAxisA=+X  BaseAlignAxisA=+Y  FollAlignAxisB=+Y  BaseAlignAxisB=+Z  RotationSequenceAxes=FollowerAxes  RotationSequence=XYX  RotationSequenceAngles=[0 0 0]  RotationSequenceAnglesUnits=deg  RotationMatrix=[1 0 0; 0 1 0; 0 0 1]  Quaternion=[1 0 0 0]
  Weld Joint : sm_lib/Joints/Weld Joint  JointMode=Normal  SenseConstraintForce=off  SenseConstraintForceX=off  SenseConstraintForceY=off  SenseConstraintForceZ=off  SenseConstraintTorque=off  SenseConstraintTorqueX=off  SenseConstraintTorqueY=off  SenseConstraintTorqueZ=off  SenseTotalForce=off  SenseTotalForceX=off  SenseTotalForceY=off  SenseTotalForceZ=off  SenseTotalTorque=off  SenseTotalTorqueX=off  SenseTotalTorqueY=off  SenseTotalTorqueZ=off  CompositeWrenchDir=FollowerOnBase  CompositeWrenchFrame=BaseFrame
  World Frame : sm_lib/Frames and Transforms/World Frame
  q1_dd : Outport
  q2_dd : Outport  Port=2
  Fn : Outport  Port=3
  X_dd : Outport  Port=4
  Y_dd : Outport  Port=5
  wires:
  Input/1 -> Simulink-PS Converter/1
  Input1/1 -> Simulink-PS Converter1/1
  PS-Simulink Converter/1 -> q1_dd/1
  PS-Simulink Converter1/1 -> q2_dd/1
  PS-Simulink Converter2/1 -> Fn/1
  PS-Simulink Converter3/1 -> X_dd/1
  PS-Simulink Converter4/1 -> Y_dd/1
  connections:
  BJ1/LConn1 -- Base/RConn1 -- WB1/RConn1
  J1L1/RConn1 -- L1J2/LConn1 -- Brick Solid1/RConn1
  Revolute Joint1/LConn1 -- L1J2/RConn1
  Brick Solid2/RConn1 -- J2L1/LConn1 -- J2L2/RConn1
  J1L1/LConn1 -- Revolute Joint/RConn1
  J2L2/LConn1 -- Revolute Joint1/RConn1
  Revolute Joint/LConn2 -- Simulink-PS Converter/RConn1
  Simulink-PS Converter1/RConn1 -- Revolute Joint1/LConn2
  Revolute Joint/RConn2 -- PS-Simulink Converter/LConn1
  PS-Simulink Converter1/LConn1 -- Revolute Joint1/RConn2
  Solver Configuration/RConn1 -- WB2/RConn1 -- WB1/LConn1 -- Mechanism Configuration/RConn1 -- World Frame/RConn1
  WB4/RConn1 -- WB2/LConn1
  J2L1/RConn1 -- Weld Joint/LConn1
  Weld Joint/RConn1 -- Cylindrical Solid/RConn1
  BJ2/RConn1 -- Revolute Joint/LConn1
  WB4/LConn1 -- Brick Solid/RConn1 -- WB3/RConn1
  Spatial Contact Force/RConn2 -- PS-Simulink Converter2/LConn1
  BJ1/RConn1 -- BJ2/LConn1
  Brick Solid3/LConn1 -- Spatial Contact Force1/LConn1 -- Spatial Contact Force/RConn1
  Cylindrical Solid/LConn1 -- Spatial Contact Force/LConn1
  Brick Solid/LConn1 -- Spatial Contact Force1/RConn1
  WB3/LConn1 -- Cartesian Joint/LConn1
  Brick Solid3/RConn1 -- Cartesian Joint/RConn1
  PS-Simulink Converter3/LConn1 -- Cartesian Joint/RConn2
  PS-Simulink Converter4/LConn1 -- Cartesian Joint/RConn3

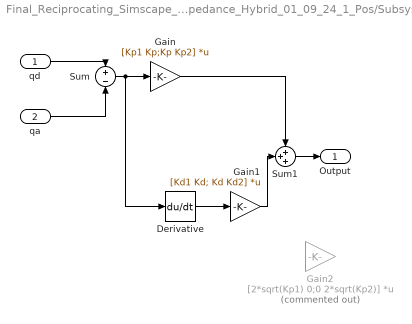
== system Final_Reciprocating_Simscape_Impedance_Hybrid_01_09_24_1_Pos/Subsystem ==
  qd : Inport
  qa : Inport  Port=2
  Derivative : Derivative
  Gain : Gain  Gain=[Kp1 Kp;Kp Kp2]  Multiplication=Matrix(K*u)
  Gain1 : Gain  Gain=[Kd1 Kd; Kd Kd2]  Multiplication=Matrix(K*u)
  Gain2 : Gain  Commented=on  Gain=[2*sqrt(Kp1) 0;0 2*sqrt(Kp2)]  Multiplication=Matrix(K*u)
  Sum : Sum  Inputs=+-
  Sum1 : Sum  Inputs=+++
  Output : Outport
  wires:
  qd/1 -> Sum/1
  qa/1 -> Sum/2
  Sum/1 -> Derivative/1, Gain/1
  Gain/1 -> Sum1/1
  Gain1/1 -> Sum1/2
  Derivative/1 -> Gain1/1
  Sum1/1 -> Output/1

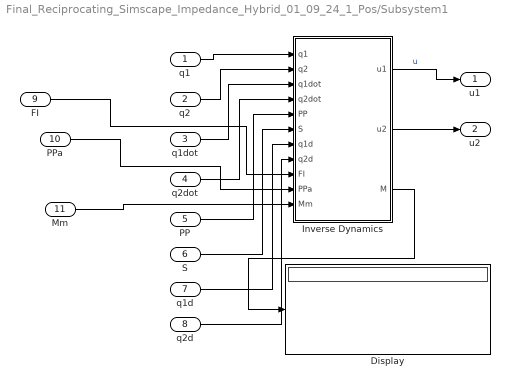
== system Final_Reciprocating_Simscape_Impedance_Hybrid_01_09_24_1_Pos/Subsystem1 ==
  q1 : Inport
  q2 : Inport  Port=2
  q1dot : Inport  Port=3
  q2dot : Inport  Port=4
  PP : Inport  Port=5
  S : Inport  Port=6
  q1d : Inport  Port=7
  q2d : Inport  Port=8
  FI : Inport  Port=9
  PPa : Inport  Port=10
  Mm : Inport  Port=11
  Display : Display
  Inverse Dynamics : MATLAB Function  TreatAsAtomicUnit=on
  u1 : Outport
  u2 : Outport  Port=2
  wires:
  q1/1 -> Inverse Dynamics/1(q1)
  q2/1 -> Inverse Dynamics/2(q2)
  q1dot/1 -> Inverse Dynamics/3(q1dot)
  q2dot/1 -> Inverse Dynamics/4(q2dot)
  PP/1 -> Inverse Dynamics/5(PP)
  S/1 -> Inverse Dynamics/6(S)
  q1d/1 -> Inverse Dynamics/7(q1d)
  q2d/1 -> Inverse Dynamics/8(q2d)
  Inverse Dynamics/1(u1) -> u1/1  "u"
  Inverse Dynamics/2(u2) -> u2/1
  FI/1 -> Inverse Dynamics/9(FI)
  PPa/1 -> Inverse Dynamics/10(PPa)
  Mm/1 -> Inverse Dynamics/11(Mm)
  Inverse Dynamics/3(M) -> Display/1

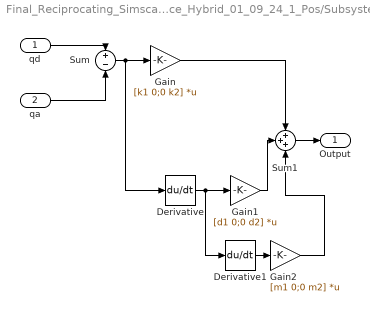
== system Final_Reciprocating_Simscape_Impedance_Hybrid_01_09_24_1_Pos/Subsystem2 ==
  qd : Inport
  qa : Inport  Port=2
  Derivative : Derivative
  Derivative1 : Derivative
  Gain : Gain  Gain=[k1 0;0 k2]  Multiplication=Matrix(K*u)
  Gain1 : Gain  Gain=[d1 0;0 d2]  Multiplication=Matrix(K*u)
  Gain2 : Gain  Gain=[m1 0;0 m2]  Multiplication=Matrix(K*u)
  Sum : Sum  Inputs=+-
  Sum1 : Sum  Inputs=+++
  Output : Outport
  wires:
  qd/1 -> Sum/1
  qa/1 -> Sum/2
  Sum/1 -> Derivative/1, Gain/1
  Gain/1 -> Sum1/1
  Gain1/1 -> Sum1/2
  Derivative/1 -> Derivative1/1, Gain1/1
  Sum1/1 -> Output/1
  Derivative1/1 -> Gain2/1
  Gain2/1 -> Sum1/3

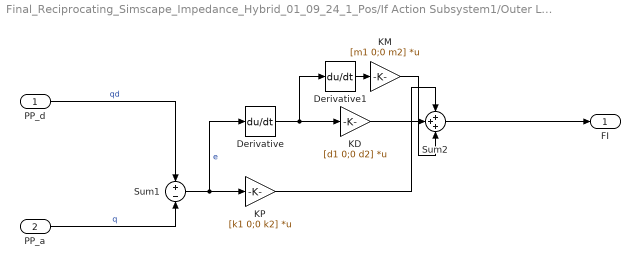
== system Final_Reciprocating_Simscape_Impedance_Hybrid_01_09_24_1_Pos/If Action Subsystem1/Outer Loop Control1 ==
  PP_d : Inport
  PP_a : Inport  Port=2
  Derivative : Derivative
  Derivative1 : Derivative
  KD : Gain  Gain=[d1 0;0 d2]  Multiplication=Matrix(K*u)
  KM : Gain  Gain=[m1 0;0 m2]  Multiplication=Matrix(K*u)
  KP : Gain  Gain=[k1 0;0 k2]  Multiplication=Matrix(K*u)
  Sum1 : Sum  Inputs=+-
  Sum2 : Sum  Inputs=+++
  FI : Outport
  wires:
  KD/1 -> Sum2/2
  KP/1 -> Sum2/1
  Sum1/1 -> Derivative/1, KP/1  "e"
  Derivative/1 -> Derivative1/1, KD/1
  PP_d/1 -> Sum1/1  "qd"
  PP_a/1 -> Sum1/2  "q"
  Sum2/1 -> FI/1
  Derivative1/1 -> KM/1
  KM/1 -> Sum2/3

== matlab function Final_Reciprocating_Simscape_Impedance_Hybrid_01_09_24_1_Pos/Subsystem1/Inverse Dynamics ==
  data: q1 input; u1 output; u2 output; q2 input; q1dot input; q2dot input; PP input; S input; q1d input; q2d input; FI input; PPa input; Mm input; M output
function [u1,u2,M] = fcn(q1,q2,q1dot,q2dot,PP,S,q1d,q2d,FI,PPa,Mm)
mo=1.8;
g=-9.81;
a1=0.5;  
a2=0.5; 
L01=0.5;
mu=0.3;
ME=1;
m1=1.56*ME;
m2=1.5288*ME;
m3=0.0490088*ME;
C1=a1/2;
C2=(m2*0.5*a2+m3*a2)/(m2+m3); 
Itot1=0.032552;
Itot2=0.0306397+2.45044e-06;
M=R_M(C1,C2,Itot1,Itot2,a1,m1,m2+m3,q2);
Cf=RCf(C2,a1,m2,q2,q1dot,q2dot);
% C = R_damp(C2,a1,m2+m3,q2,q1dot,q2dot);
Gr= R_Gra(C1,C2,a1,m1,m2+m3,g,q1,q2);
Jac = R_Jac(a1,a2,q1,q2);
Jacd = R_Jac(a1,a2,q1d,q2d);
Jd=R_Jd(a1,a2,q1,q2,q1d,q2d);
% u=M*inv(Jacd)*PP(1:2)+ Cf+Gr+inv(Jacd)*S+Jacd'*FI;
% u=M*inv(Jacd)*PP(1:2)-M*inv(Jacd)*Jd*[q1d;q2d]+ Cf+Gr+inv(Jacd)*S;
% u=M*inv(Jac)*PP(1:2)-M*inv(Jac)*Jd*[q1;q2]+ Cf+Gr+inv(Jac)*S; 

% u=M*inv(Jac)*PP(1:2)-Jac'*S;
% u=Jacd'*S;
% Mm=M;
Fa=Mm*(PP(1:2)-PPa(1:2))+S;
u=M*inv(Jac)*(PP(1:2)-Jd*[q1;q2]+inv(Mm)* S)+Cf+Gr+Jac'*(M*inv(Mm)-eye(2))*Fa; 
u1=u(1);
u2=u(2);

== matlab function Final_Reciprocating_Simscape_Impedance_Hybrid_01_09_24_1_Pos/MATLAB Function ==
  data: Fcd output; Pdd input; Fn output; Fna input
function [Fcd, Fn ]= fcn(Pdd,Fna)

mus=0.3;
mo=1.8;
g=-9.81;
mu=0.5;
xdd=Pdd(1);
if Fna==0
    Fcd=[0;0];Fn=0;
else
Fcd = R_Fcd(g,mo,mu,mus,xdd)
Ft=Fcd(1);
Fn=Fcd(2);
end

== matlab function Final_Reciprocating_Simscape_Impedance_Hybrid_01_09_24_1_Pos/Forward  Kinemtics ==
  data: q1 input; PP output; q2 input
function PP = fcn(q1,q2)
a1=0.5;
a2=0.5;
L01=0.5;
r=0.01;
PP=R_EQ1(L01,a1,a2,r,q1,q2);
